simulink subsystem "climb_control_PI"  (R2021a)
settings: Solver=VariableStepAuto  StartTime=0.0  StopTime=10.0  RelTol=1e-3
undefined symbols (not defined in the file or in its folder): C_climb, DiscIntNeverNeededParam, g, T_max
settings Model: Creator=EpEp  LastModifiedBy=EpEp

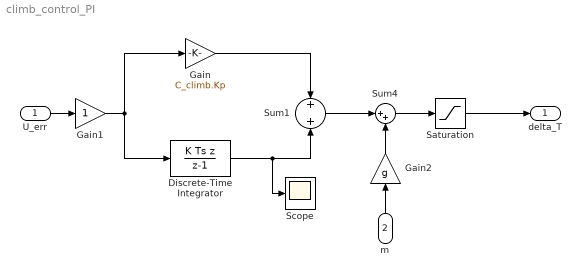
== system climb_control_PI ==
  U_err : Inport
  m : Inport  Port=2
  Discrete-Time Integrator : DiscreteIntegrator  IntegratorMethod=Integration: Backward Euler  gainval=C_climb.Ki  SampleTime=C_climb.Ts  LimitOutput=on  UpperSaturationLimit=500  LowerSaturationLimit=-80  ICPrevOutput=DiscIntNeverNeededParam  ICPrevScaledInput=DiscIntNeverNeededParam
  Gain : Gain  Gain=C_climb.Kp
  Gain1 : Gain
  Gain2 : Gain  Gain=g
  Saturation : Saturate  UpperLimit=T_max  LowerLimit=0
  Scope : Scope
  Sum1 : Sum  Inputs=+|+
  Sum4 : Sum  Inputs=|++
  delta_T : Outport
  wires:
  Gain/1 -> Sum1/1
  Discrete-Time Integrator/1 -> Sum1/2, Scope/1
  Sum1/1 -> Sum4/1
  U_err/1 -> Gain1/1
  Gain1/1 -> Gain/1, Discrete-Time Integrator/1
  Gain2/1 -> Sum4/2
  Sum4/1 -> Saturation/1
  Saturation/1 -> delta_T/1
  m/1 -> Gain2/1
